simulink model "stack_parameters_standalone"  (R2023a)
settings: Solver=VariableStepAuto  StartTime=0.0  StopTime=10.0  RelTol=1e-3
settings Model: Creator=adrian.taveras  LastModifiedBy=adrian.taveras

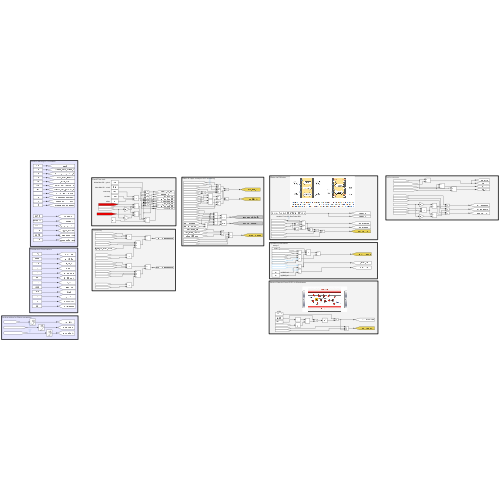
[thumbnail: Simulink's stored preview of the top-level diagram]
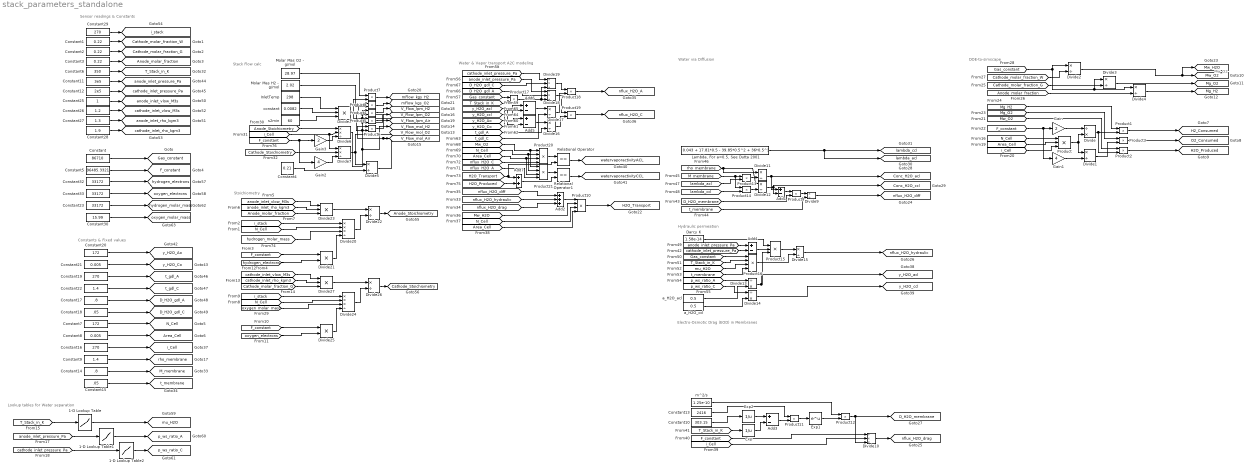
== system stack_parameters_standalone ==
  note: Lookup tables for Water separation
  note: Hydraulic permeation
  note: Electro-Osmotic Drag (EOD) in Membranes
  note: DOE-to-simscape
  note: Water via Diffusion
  note: Mw_O2
  note: Stack Flow calc
  note: Constants & Fixed values
  note: Sensor readings & Constants
  note: Water & Vapor transport A2C modeling
  note: Stoichiometry
  1-D Lookup Table : Lookup_n-D  NumberOfTableDimensions=1  BreakpointsForDimension1=[-5:5]  Table=tanh([-5:5])  InternalRulePriority=Speed  RndMeth=Simplest
  1-D Lookup Table1 : Lookup_n-D  NumberOfTableDimensions=1  BreakpointsForDimension1=[-5:5]  Table=tanh([-5:5])  InternalRulePriority=Speed  RndMeth=Simplest
  1-D Lookup Table2 : Lookup_n-D  NumberOfTableDimensions=1  BreakpointsForDimension1=[-5:5]  Table=tanh([-5:5])  InternalRulePriority=Speed  RndMeth=Simplest
  Add{1,3..6} (5 alike) : Sum  Inputs=+-
  Add2 : Sum  Inputs=+++
  Add7 : Sum
  Constant : Constant  Value=86710
  Constant1 : Constant  Value=0.22
  Constant10 : Constant  Value=303.15
  Constant11 : Constant  Value=3e5
  Constant12 : Constant  Value=2e5
  Constant13 : Constant  Value=2416
  Constant14 : Constant  Value=.8
  Constant15 : Constant  Value=.05
  Constant16 : Constant  Value=270
  Constant17 : Constant  Value=.8
  Constant18 : Constant  Value=.05
  Constant19 : Constant  Value=270
  Constant2 : Constant  Value=0.22
  Constant20 : Constant  Value=172
  Constant21 : Constant  Value=0.005
  Constant22 : Constant  Value=1.4
  Constant23 : Constant  Value=33172
  Constant25 : Constant
  Constant26 : Constant  Value=1.2
  Constant27 : Constant  Value=1.3
  Constant28 : Constant  Value=1.9
  Constant29 : Constant  Value=270
  Constant3 : Constant  Value=0.22
  Constant30 : Constant  Value=15.99
  Constant32 : Constant  Value=33172
  Constant33 : Constant  Value=33172
  Constant4 : Constant  Value=0.21
  Constant5 : Constant  Value=96485.3321
  Constant6 : Constant  Value=350
  Constant7 : Constant  Value=172
  Constant8 : Constant  Value=0.005
  Constant9 : Constant  Value=1.4
  Darcy K : Constant  Value=1.58e-14
  Divide : Product  Inputs=/*
  Divide{1..5,9,11..12,15..17,22,26} (13 alike) : Product  Inputs=*/
  Divide10 : Product  Inputs=/**
  Divide13 : Product  Inputs=/*
  Divide14 : Product  Inputs=/*
  Divide{6..7,18..19} (4 alike) : Product  Inputs=**/
  Divide20 : Product  Inputs=***/
  Divide21 : Product  Inputs=**
  Divide23 : Product  Inputs=***
  Divide24 : Product  Inputs=***/
  Divide25 : Product  Inputs=**
  Divide27 : Product  Inputs=***
  Divide8 : Product  Inputs=***
  Exp : Math  Operator=reciprocal
  Exp1 : Math
  Exp2 : Math  Operator=reciprocal
  Gain : Gain  Gain=2
  Gain1 : Gain  Gain=4
  Gain2 : Gain  Gain=4
  Gain3 : Gain  Gain=2
  InletTemp : Constant  Value=298
  "Lambda, For a=0.5, See Dutta 2001" : Constant  Value=0.043 + 17.81*0.5 - 39.85*0.5^2 + 36*0.5^3
  Molar Mas H2 -  g/mol : Constant  Value=2.02
  "Molar Mas O2 -  g/mol " : Constant  Value=28.97
  Product : Product  Inputs=3
  Product{1..9,11..14,17..19} (16 alike) : Product
  Product{10,16,20..21} (4 alike) : Product  Inputs=4
  Product15 : Product  Inputs=3
  Relational Operator : RelationalOperator  Operator===  OutDataTypeStr=boolean  RndMeth=Simplest  InputSameDT=off
  Relational Operator1 : RelationalOperator  Operator===  OutDataTypeStr=boolean  RndMeth=Simplest  InputSameDT=off
  a_H2O_acl : Constant  Value=0.5
  a_H2O_ccl : Constant  Value=0.5
  constant : Constant  Value=0.0082
  m^2/s : Constant  Value=1.25e-10
  s2min : Constant  Value=60
  tag scope: Anode_Stoichiometry=global, Anode_molar_fraction=global, Area_Cell=global, Cathode_Stoichiometry=global, Cathode_molar_fraction_G=global, Cathode_molar_fraction_W=global, Conc_H2O_acl=global, Conc_H2O_ccl=global, D_H2O_gdl_A=global, D_H2O_gdl_C=global, D_H2O_membrane=global, F_constant=global, Gas_constant=global, H2O_Produced=global, H2O_Transport=global, H2_Consumed=global, M_membrane=global, Mg_H2=global, Mg_O2=global, Mw_H2O=global, Mw_O2=global, N_Cell=global, O2_Consumed=global, T_Stack_in_K=global, V_Flow_lpm_Air=global, V_Flow_lpm_H2=global, V_Flow_lpm_O2=global, V_Flow_mol_Air=global, V_Flow_mol_H2=global, V_Flow_mol_O2=global, anode_inlet_pressure_Pa=global, anode_inlet_rho_kgm3=global, anode_inlet_vlow_M3s=global, cathode_inlet_pressure_Pa=global, cathode_inlet_rho_kgm3=global, cathode_inlet_vlow_M3s=global, hydrogen_electrons=global, hydrogen_molar_mass=global, i_Cell=global, i_stack=global, lambda_acl=global, lambda_ccl=global, mFlow_kgs_H2=global, mFlow_kgs_O2=global, mu_H2O=global, nflux_H2O_A=global, nflux_H2O_C=global, nflux_H2O_diff=global, nflux_H2O_drag=global, nflux_H2O_hydraulic=global, oxygen_electrons=global, oxygen_molar_mass=global, p_ws_ratio_A=global, p_ws_ratio_C=global, rho_membrane=global, t_gdl_A=global, t_gdl_C=global, t_membrane=global, watervaporactivityACL=global, watervaporactivityCCL=global, y_H2O_Ao=global, y_H2O_Co=global, y_H2O_acl=global, y_H2O_ccl=global
  wires:
  Constant2/1 -> [Cathode_molar_fraction_G]
  Constant3/1 -> [Anode_molar_fraction]
  Constant/1 -> [Gas_constant]
  Constant15/1 -> [t_membrane]
  Constant14/1 -> [M_membrane]
  [N_Cell] -> Product10/3
  Gain3/1 -> Divide6/3
  [rho_membrane] -> Divide11/1, Divide12/1
  [F_constant] -> Divide10/1
  Darcy K/1 -> Product15/1
  [y_H2O_Co] -> Add6/2
  [nflux_H2O_drag] -> Add2/3
  Add3/1 -> Product11/2
  [y_H2O_acl] -> Add5/2
  [H2O_Produced] -> Add7/2
  Add7/1 -> Relational Operator1/2
  Divide17/1 -> Product18/2
  [Area_Cell] -> Product10/4
  Divide11/1 -> Add1/1, [Conc_H2O_acl]
  Product/1 -> Divide1/1, Divide/2
  Constant10/1 -> Exp2/1
  [i_Cell] -> Divide10/2
  Add1/1 -> Product9/1
  [mu_H2O] -> Product16/3
  Exp/1 -> Add3/2
  Product12/1 -> [D_H2O_membrane], Divide10/3
  Divide14/1 -> [y_H2O_ccl]
  [Area_Cell] -> Product/2
  Divide10/1 -> [nflux_H2O_drag]
  Divide/1 -> Product1/2, Product2/2
  Product21/1 -> Relational Operator1/1
  [Area_Cell] -> Product20/3, Product21/3
  Product11/1 -> Exp1/1
  Gain1/1 -> Divide1/2
  [T_Stack_in_K] -> Product16/2
  Product7/1 -> [mFlow_kgs_H2]
  [H2O_Transport] -> Add7/1, Relational Operator/2
  [T_Stack_in_K] -> Exp/1
  [i_Cell] -> Divide7/1, Divide6/2
  Product4/1 -> [V_Flow_lpm_H2]
  s2min/1 -> Divide8/3
  [D_H2O_membrane] -> Product9/2
  Exp2/1 -> Add3/1
  Divide13/1 -> Product15/3, [y_H2O_acl]
  Product13/1 -> Divide11/2
  Product14/1 -> Divide12/2
  Product17/1 -> Divide18/3, Divide19/3
  Add5/1 -> Divide16/1
  [lambda_acl] -> Product13/2
  m^2/s/1 -> Product12/1
  Divide6/1 -> Product4/1, [V_Flow_mol_H2]
  Product1/1 -> [H2_Consumed]
  [N_Cell] -> Product20/2, Product21/2
  Constant17/1 -> [D_H2O_gdl_A]
  [anode_inlet_pressure_Pa] -> Add4/1
  [Gas_constant] -> Divide2/1, Divide4/1, Divide3/1
  Divide9/1 -> [nflux_H2O_diff]
  Constant9/1 -> [rho_membrane]
  Constant19/1 -> [t_gdl_A]
  Constant6/1 -> [T_Stack_in_K]
  Constant7/1 -> [N_Cell]
  Constant8/1 -> [Area_Cell]
  Constant5/1 -> [F_constant]
  Constant21/1 -> [y_H2O_Co]
  Product16/1 -> Divide15/2
  Product9/1 -> Divide9/1
  Product8/1 -> [mFlow_kgs_O2]
  [anode_inlet_pressure_Pa] -> Divide18/1
  Product19/1 -> [nflux_H2O_C]
  [Mw_O2] -> Product2/1
  Constant12/1 -> [cathode_inlet_pressure_Pa]
  Add4/1 -> Product15/2
  Divide19/1 -> Product18/1
  [Cathode_molar_fraction_W] -> Divide2/2
  [t_membrane] -> Divide9/2
  [nflux_H2O_C] -> Product20/4
  Divide3/1 -> [Mg_O2]
  [nflux_H2O_hydraulic] -> Add2/2
  [Gas_constant] -> Product16/1
  [t_gdl_A] -> Divide16/2
  Gain/1 -> Divide/1
  Add6/1 -> Divide17/1
  [t_gdl_C] -> Divide17/2
  Divide18/1 -> Product19/1
  [nflux_H2O_A] -> Product21/4
  [F_constant] -> Gain3/1, Gain2/1
  Divide16/1 -> Product19/2
  [y_H2O_Ao] -> Add5/1
  [F_constant] -> Gain1/1, Gain/1
  InletTemp/1 -> Divide8/1
  Constant4/1 -> Divide5/2
  [M_membrane] -> Product14/1, Product13/1
  Constant20/1 -> [y_H2O_Ao]
  [Anode_Stoichiometry] -> Divide6/1
  [Anode_molar_fraction] -> Divide4/2
  [Cathode_molar_fraction_G] -> Divide3/2
  Divide15/1 -> [nflux_H2O_hydraulic]
  a_H2O_acl/1 -> Divide13/2
  [i_Cell] -> Product/3
  Product6/1 -> [V_Flow_lpm_Air]
  Exp1/1 -> Product12/2
  [p_ws_ratio_A] -> Divide13/1
  [p_ws_ratio_C] -> Divide14/1
  Constant16/1 -> [i_Cell]
  [Mg_H2] -> Product1/1
  Product15/1 -> Divide15/1
  Divide1/1 -> Product3/2
  Constant11/1 -> [anode_inlet_pressure_Pa]
  Molar Mas H2 -  g/mol/1 -> Product8/2
  [Mw_H2O] -> Product10/2
  Product2/1 -> [H2O_Produced]
  Product3/1 -> [O2_Consumed]
  "Lambda, For a=0.5, See Dutta 2001"/1 -> [lambda_ccl], [lambda_acl]
  Divide2/1 -> [Mw_O2], [Mw_H2O]
  Product5/1 -> [V_Flow_lpm_O2]
  Divide12/1 -> [Conc_H2O_ccl], Add1/2
  [Mg_O2] -> Product3/1
  [cathode_inlet_pressure_Pa] -> Add4/2
  Product18/1 -> [nflux_H2O_A]
  [lambda_ccl] -> Product14/2
  constant/1 -> Divide8/2
  Divide5/1 -> [V_Flow_mol_Air], Product6/1
  a_H2O_ccl/1 -> Divide14/2
  Constant22/1 -> [t_gdl_C]
  [T_Stack_in_K] -> Product17/2
  [Cathode_Stoichiometry] -> Divide7/2
  [N_Cell] -> Product/1
  Gain2/1 -> Divide7/3
  [D_H2O_gdl_C] -> Divide19/2
  [cathode_inlet_pressure_Pa] -> Divide19/1
  [y_H2O_ccl] -> Add6/1
  [D_H2O_gdl_A] -> Divide18/2
  [nflux_H2O_diff] -> Add2/1
  "Molar Mas O2 -  g/mol "/1 -> Product7/1
  Relational Operator/1 -> [watervaporactivityACL]
  Divide4/1 -> [Mg_H2]
  [Gas_constant] -> Product17/1
  Divide7/1 -> Divide5/1, Product5/1, Product7/2, [V_Flow_mol_O2]
  Product10/1 -> [H2O_Transport]
  Add2/1 -> Product10/1
  Relational Operator1/1 -> [watervaporactivityCCL]
  Constant18/1 -> [D_H2O_gdl_C]
  Divide8/1 -> Product6/2, Product5/2, Product4/2, Product8/1
  Constant13/1 -> Product11/1
  [t_membrane] -> Product16/4
  Product20/1 -> Relational Operator/1
  Constant1/1 -> [Cathode_molar_fraction_W]
  [Mw_O2] -> Product20/1, Product21/1
  [i_stack] -> Divide20/1
  [N_Cell] -> Divide20/2
  [hydrogen_molar_mass] -> Divide20/3
  [F_constant] -> Divide21/1
  [hydrogen_electrons] -> Divide21/2
  Divide21/1 -> Divide20/4
  Divide20/1 -> Divide22/2
  Constant25/1 -> [anode_inlet_vlow_M3s]
  Constant26/1 -> [cathode_inlet_vlow_M3s]
  Constant27/1 -> [anode_inlet_rho_kgm3]
  Constant28/1 -> [cathode_inlet_rho_kgm3]
  Constant29/1 -> [i_stack]
  [Anode_molar_fraction] -> Divide23/3
  [anode_inlet_rho_kgm3] -> Divide23/2
  [anode_inlet_vlow_M3s] -> Divide23/1
  Divide23/1 -> Divide22/1
  Divide22/1 -> [Anode_Stoichiometry]
  Divide26/1 -> [Cathode_Stoichiometry]
  Divide27/1 -> Divide26/1
  [cathode_inlet_vlow_M3s] -> Divide27/1
  [cathode_inlet_rho_kgm3] -> Divide27/2
  [Cathode_molar_fraction_G] -> Divide27/3
  Divide24/1 -> Divide26/2
  Divide25/1 -> Divide24/4
  [oxygen_electrons] -> Divide25/2
  [F_constant] -> Divide25/1
  [oxygen_molar_mass] -> Divide24/3
  [N_Cell] -> Divide24/2
  [i_stack] -> Divide24/1
  Constant32/1 -> [hydrogen_electrons]
  Constant33/1 -> [oxygen_electrons]
  [T_Stack_in_K] -> 1-D Lookup Table/1
  [anode_inlet_pressure_Pa] -> 1-D Lookup Table1/1
  [cathode_inlet_pressure_Pa] -> 1-D Lookup Table2/1
  1-D Lookup Table/1 -> [mu_H2O]
  1-D Lookup Table1/1 -> [p_ws_ratio_A]
  1-D Lookup Table2/1 -> [p_ws_ratio_C]
  Constant30/1 -> [oxygen_molar_mass]
  Constant23/1 -> [hydrogen_molar_mass]
